simulink model "test"  (R2014a)
settings: Solver=ode45  StartTime=0.0  StopTime=20  MaxStep=0.001  RelTol=1e-3
settings Model: Creator=Etienne  LastModifiedBy=Etienne

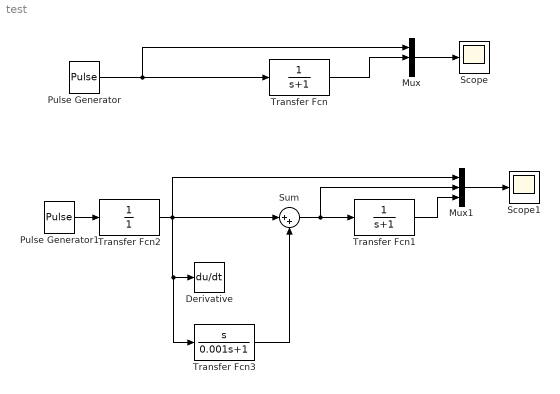
== system test ==
  Derivative : Derivative
  Mux : Mux  Inputs=3
  Mux1 : Mux  Inputs=3
  Pulse Generator : DiscretePulseGenerator  PulseType=Time based  Period=5  PulseWidth=50
  Pulse Generator1 : DiscretePulseGenerator  PulseType=Time based  Period=5  PulseWidth=50
  Scope : Scope
  Scope1 : Scope
      settings: MaxDataPoints=500000
  Sum : Sum  Inputs=|++
  Transfer Fcn : TransferFcn  Denominator=[1 1]
  Transfer Fcn1 : TransferFcn  Denominator=[1 1]
  Transfer Fcn2 : TransferFcn  Denominator=[.00 1]
  Transfer Fcn3 : TransferFcn  Numerator=[1 0]  Denominator=[0.001 1]
  wires:
  Mux/1 -> Scope/1
  Transfer Fcn/1 -> Mux/2
  Pulse Generator/1 -> Transfer Fcn/1, Mux/1
  Mux1/1 -> Scope1/1
  Pulse Generator1/1 -> Transfer Fcn2/1
  Sum/1 -> Mux1/2, Transfer Fcn1/1
  Transfer Fcn2/1 -> Mux1/1, Sum/1, Transfer Fcn3/1, Derivative/1
  Transfer Fcn3/1 -> Sum/2
  Transfer Fcn1/1 -> Mux1/3
